simulink model "ALU_zipVer_Updated"  (R2023a)
settings: Solver=VariableStepAuto  StartTime=0.0  StopTime=10.0  RelTol=1e-3
settings Model: Creator=serge  LastModifiedBy=serge

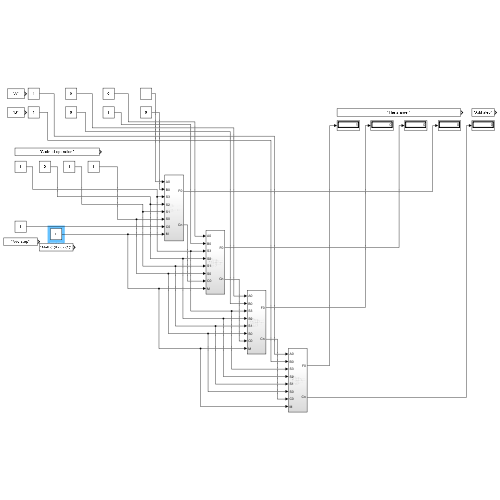
[thumbnail: Simulink's stored preview of the top-level diagram]
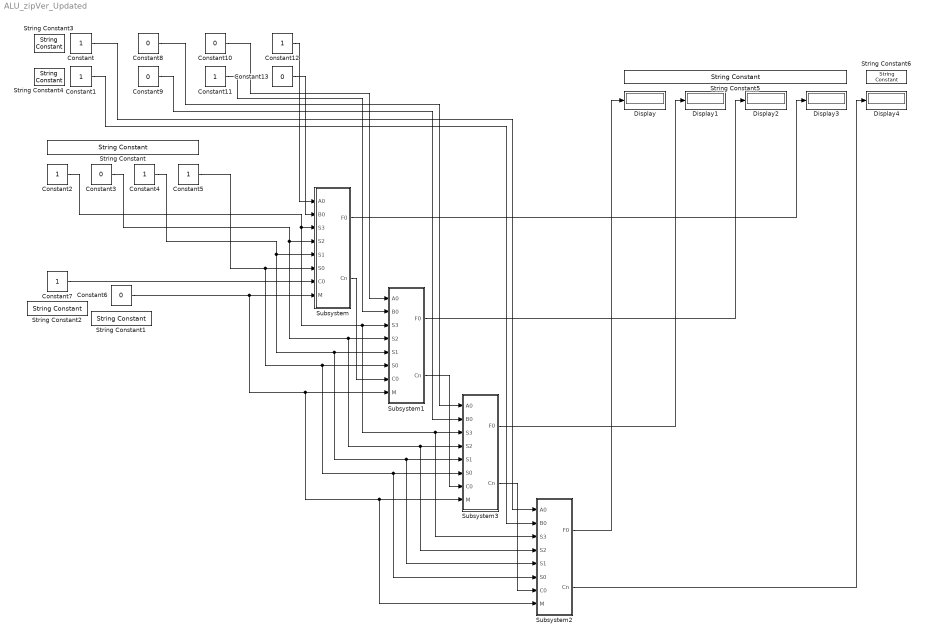
== system ALU_zipVer_Updated ==
  Constant{,1..2,4..5,7,11..12} (8 alike) : Constant
  Constant{3,6,8..10,13} (6 alike) : Constant  Value=0
  Display{,1..4} (5 alike) : Display
  String Constant : StringConstant  String="\"Code of operation\""
  String Constant1 : StringConstant  String="\"Math(0)/Logic(1)\""
  String Constant2 : StringConstant  String="\"Add step\""
  String Constant3 : StringConstant  String="\"A\""
  String Constant4 : StringConstant  String="\"B\""
  String Constant5 : StringConstant  String="\"The answer\""
  String Constant6 : StringConstant  String="\"Add step\""
  Subsystem : Subsystem
  Subsystem1 : Subsystem
  Subsystem2 : Subsystem
  Subsystem3 : Subsystem
  wires:
  Constant/1 -> Subsystem2/1(A0)
  Constant1/1 -> Subsystem2/2(B0)
  Constant3/1 -> Subsystem1/4(S2), Subsystem2/4(S2), Subsystem3/4(S2), Subsystem/4(S2)
  Constant4/1 -> Subsystem1/5(S1), Subsystem2/5(S1), Subsystem3/5(S1), Subsystem/5(S1)
  Constant5/1 -> Subsystem2/6(S0), Subsystem3/6(S0), Subsystem1/6(S0), Subsystem/6(S0)
  Constant6/1 -> Subsystem1/8(M), Subsystem2/8(M), Subsystem3/8(M), Subsystem/8(M)
  Constant7/1 -> Subsystem/7(C0)
  Subsystem/2(Cn) -> Subsystem1/7(C0)
  Subsystem1/2(Cn) -> Subsystem3/7(C0)
  Subsystem3/2(Cn) -> Subsystem2/7(C0)
  Constant2/1 -> Subsystem1/3(S3), Subsystem2/3(S3), Subsystem3/3(S3), Subsystem/3(S3)
  Constant8/1 -> Subsystem3/1(A0)
  Constant9/1 -> Subsystem3/2(B0)
  Constant10/1 -> Subsystem1/1(A0)
  Constant11/1 -> Subsystem1/2(B0)
  Constant13/1 -> Subsystem/2(B0)
  Constant12/1 -> Subsystem/1(A0)
  Subsystem2/2(Cn) -> Display4/1
  Subsystem2/1(F0) -> Display/1
  Subsystem3/1(F0) -> Display1/1
  Subsystem1/1(F0) -> Display2/1
  Subsystem/1(F0) -> Display3/1

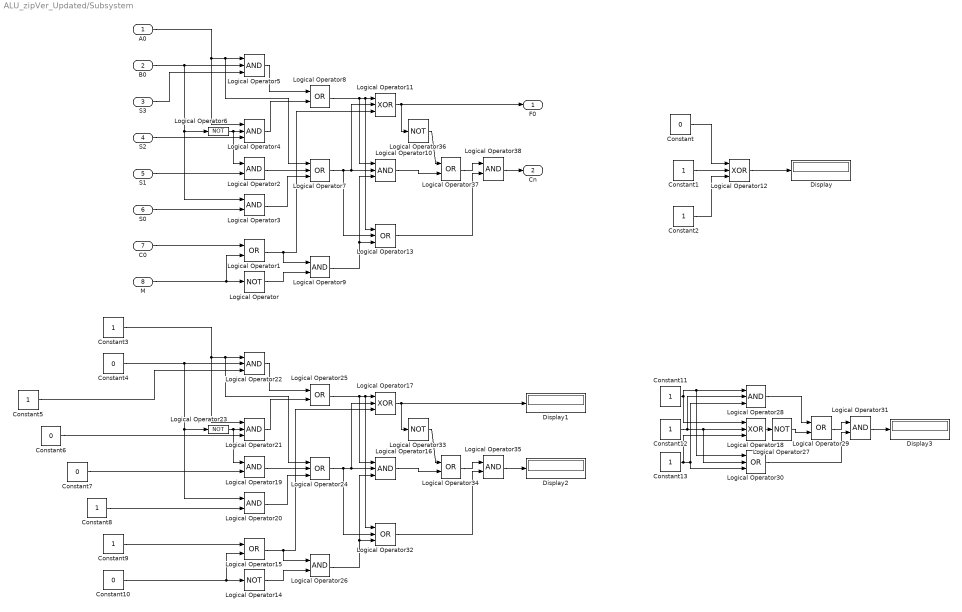
== system ALU_zipVer_Updated/Subsystem ==
  A0 : Inport
  B0 : Inport  Port=2
  S3 : Inport  Port=3
  S2 : Inport  Port=4
  S1 : Inport  Port=5
  S0 : Inport  Port=6
  C0 : Inport  Port=7
  M : Inport  Port=8
  Constant{,4,6..7,10} (5 alike) : Constant  Value=0
  Constant{1..3,5,8..9,11..13} (9 alike) : Constant
  Display{,1..3} (4 alike) : Display
  Logical Operator{,6,14,23} (4 alike) : Logic  Operator=NOT  AllPortsSameDT=off  OutDataTypeStr=boolean
  Logical Operator{1,8,15,25,29,34,37} (7 alike) : Logic  Operator=OR  AllPortsSameDT=off  OutDataTypeStr=boolean
  Logical Operator{4..5,10,16,21..22,28} (7 alike) : Logic  Inputs=3  AllPortsSameDT=off  OutDataTypeStr=boolean
  Logical Operator{11..12,17..18} (4 alike) : Logic  Operator=XOR  Inputs=3  AllPortsSameDT=off  OutDataTypeStr=boolean
  Logical Operator{7,13,24,30,32} (5 alike) : Logic  Operator=OR  Inputs=3  AllPortsSameDT=off  OutDataTypeStr=boolean
  Logical Operator{2..3,9,19..20,26,31,35,38} (9 alike) : Logic  AllPortsSameDT=off  OutDataTypeStr=boolean
  Logical Operator27 : Logic  Operator=NOT  Inputs=3  AllPortsSameDT=off  OutDataTypeStr=boolean
  Logical Operator33 : Logic  Operator=NOT  Inputs=3  AllPortsSameDT=off  OutDataTypeStr=boolean
  Logical Operator36 : Logic  Operator=NOT  Inputs=3  AllPortsSameDT=off  OutDataTypeStr=boolean
  F0 : Outport
  Cn : Outport  Port=2
  wires:
  S0/1 -> Logical Operator3/2
  Logical Operator6/1 -> Logical Operator2/1, Logical Operator4/2
  B0/1 -> Logical Operator5/2, Logical Operator6/1, Logical Operator3/1
  Logical Operator5/1 -> Logical Operator8/1
  Logical Operator/1 -> Logical Operator9/2
  M/1 -> Logical Operator/1, Logical Operator1/2
  A0/1 -> Logical Operator7/1, Logical Operator5/1, Logical Operator4/1
  S3/1 -> Logical Operator5/3
  C0/1 -> Logical Operator1/1
  Logical Operator4/1 -> Logical Operator8/2
  Logical Operator2/1 -> Logical Operator7/2
  Logical Operator3/1 -> Logical Operator7/3
  S1/1 -> Logical Operator2/2
  S2/1 -> Logical Operator4/3
  Constant/1 -> Logical Operator12/1
  Constant1/1 -> Logical Operator12/2
  Constant2/1 -> Logical Operator12/3
  Logical Operator12/1 -> Display/1
  Logical Operator25/1 -> Logical Operator16/1, Logical Operator32/1, Logical Operator17/1
  Logical Operator22/1 -> Logical Operator25/1
  Logical Operator21/1 -> Logical Operator25/2
  Constant6/1 -> Logical Operator21/3
  Constant9/1 -> Logical Operator15/1
  Logical Operator14/1 -> Logical Operator26/2
  Logical Operator26/1 -> Logical Operator32/3, Logical Operator16/3
  Constant3/1 -> Logical Operator24/1, Logical Operator22/1, Logical Operator21/1
  Constant4/1 -> Logical Operator22/2, Logical Operator23/1, Logical Operator20/1
  Logical Operator15/1 -> Logical Operator26/1, Logical Operator17/3
  Constant10/1 -> Logical Operator14/1, Logical Operator15/2
  Logical Operator24/1 -> Logical Operator32/2, Logical Operator17/2, Logical Operator16/2
  Logical Operator19/1 -> Logical Operator24/2
  Logical Operator16/1 -> Logical Operator34/2
  Constant8/1 -> Logical Operator20/2
  Logical Operator23/1 -> Logical Operator19/1, Logical Operator21/2
  Constant5/1 -> Logical Operator22/3
  Constant7/1 -> Logical Operator19/2
  Logical Operator20/1 -> Logical Operator24/3
  Logical Operator17/1 -> Logical Operator33/1, Display1/1
  Constant11/1 -> Logical Operator30/1, Logical Operator28/1, Logical Operator18/1
  Constant12/1 -> Logical Operator28/2, Logical Operator30/2, Logical Operator18/2
  Constant13/1 -> Logical Operator30/3, Logical Operator28/3, Logical Operator18/3
  Logical Operator18/1 -> Logical Operator27/1
  Logical Operator27/1 -> Logical Operator29/2
  Logical Operator28/1 -> Logical Operator29/1
  Logical Operator29/1 -> Logical Operator31/1
  Logical Operator30/1 -> Logical Operator31/2
  Logical Operator31/1 -> Display3/1
  Logical Operator33/1 -> Logical Operator34/1
  Logical Operator34/1 -> Logical Operator35/1
  Logical Operator32/1 -> Logical Operator35/2
  Logical Operator35/1 -> Display2/1
  Logical Operator8/1 -> Logical Operator10/1, Logical Operator13/1, Logical Operator11/1
  Logical Operator38/1 -> Cn/1
  Logical Operator10/1 -> Logical Operator37/2
  Logical Operator36/1 -> Logical Operator37/1
  Logical Operator37/1 -> Logical Operator38/1
  Logical Operator13/1 -> Logical Operator38/2
  Logical Operator11/1 -> F0/1, Logical Operator36/1
  Logical Operator1/1 -> Logical Operator11/3, Logical Operator9/1
  Logical Operator7/1 -> Logical Operator13/2, Logical Operator11/2, Logical Operator10/2
  Logical Operator9/1 -> Logical Operator13/3, Logical Operator10/3

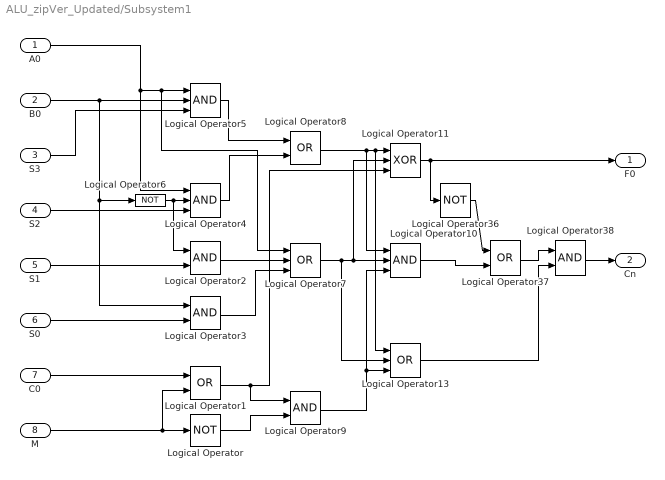
== system ALU_zipVer_Updated/Subsystem1 ==
  A0 : Inport
  B0 : Inport  Port=2
  S3 : Inport  Port=3
  S2 : Inport  Port=4
  S1 : Inport  Port=5
  S0 : Inport  Port=6
  C0 : Inport  Port=7
  M : Inport  Port=8
  Logical Operator : Logic  Operator=NOT  AllPortsSameDT=off  OutDataTypeStr=boolean
  Logical Operator1 : Logic  Operator=OR  AllPortsSameDT=off  OutDataTypeStr=boolean
  Logical Operator10 : Logic  Inputs=3  AllPortsSameDT=off  OutDataTypeStr=boolean
  Logical Operator11 : Logic  Operator=XOR  Inputs=3  AllPortsSameDT=off  OutDataTypeStr=boolean
  Logical Operator13 : Logic  Operator=OR  Inputs=3  AllPortsSameDT=off  OutDataTypeStr=boolean
  Logical Operator{2..3,9,38} (4 alike) : Logic  AllPortsSameDT=off  OutDataTypeStr=boolean
  Logical Operator36 : Logic  Operator=NOT  Inputs=3  AllPortsSameDT=off  OutDataTypeStr=boolean
  Logical Operator37 : Logic  Operator=OR  AllPortsSameDT=off  OutDataTypeStr=boolean
  Logical Operator4 : Logic  Inputs=3  AllPortsSameDT=off  OutDataTypeStr=boolean
  Logical Operator5 : Logic  Inputs=3  AllPortsSameDT=off  OutDataTypeStr=boolean
  Logical Operator6 : Logic  Operator=NOT  AllPortsSameDT=off  OutDataTypeStr=boolean
  Logical Operator7 : Logic  Operator=OR  Inputs=3  AllPortsSameDT=off  OutDataTypeStr=boolean
  Logical Operator8 : Logic  Operator=OR  AllPortsSameDT=off  OutDataTypeStr=boolean
  F0 : Outport
  Cn : Outport  Port=2
  wires:
  Logical Operator2/1 -> Logical Operator7/2
  Logical Operator4/1 -> Logical Operator8/2
  S2/1 -> Logical Operator4/3
  Logical Operator5/1 -> Logical Operator8/1
  Logical Operator36/1 -> Logical Operator37/1
  Logical Operator13/1 -> Logical Operator38/2
  Logical Operator37/1 -> Logical Operator38/1
  C0/1 -> Logical Operator1/1
  Logical Operator/1 -> Logical Operator9/2
  Logical Operator8/1 -> Logical Operator10/1, Logical Operator13/1, Logical Operator11/1
  Logical Operator7/1 -> Logical Operator13/2, Logical Operator11/2, Logical Operator10/2
  Logical Operator11/1 -> F0/1, Logical Operator36/1
  Logical Operator9/1 -> Logical Operator13/3, Logical Operator10/3
  A0/1 -> Logical Operator7/1, Logical Operator5/1, Logical Operator4/1
  B0/1 -> Logical Operator5/2, Logical Operator6/1, Logical Operator3/1
  Logical Operator1/1 -> Logical Operator11/3, Logical Operator9/1
  M/1 -> Logical Operator/1, Logical Operator1/2
  S0/1 -> Logical Operator3/2
  Logical Operator10/1 -> Logical Operator37/2
  Logical Operator6/1 -> Logical Operator2/1, Logical Operator4/2
  S3/1 -> Logical Operator5/3
  S1/1 -> Logical Operator2/2
  Logical Operator3/1 -> Logical Operator7/3
  Logical Operator38/1 -> Cn/1

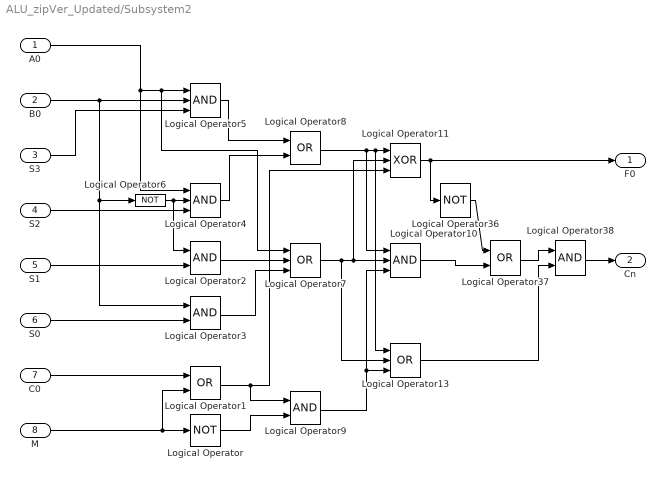
== system ALU_zipVer_Updated/Subsystem2 ==
  A0 : Inport
  B0 : Inport  Port=2
  S3 : Inport  Port=3
  S2 : Inport  Port=4
  S1 : Inport  Port=5
  S0 : Inport  Port=6
  C0 : Inport  Port=7
  M : Inport  Port=8
  Logical Operator : Logic  Operator=NOT  AllPortsSameDT=off  OutDataTypeStr=boolean
  Logical Operator1 : Logic  Operator=OR  AllPortsSameDT=off  OutDataTypeStr=boolean
  Logical Operator10 : Logic  Inputs=3  AllPortsSameDT=off  OutDataTypeStr=boolean
  Logical Operator11 : Logic  Operator=XOR  Inputs=3  AllPortsSameDT=off  OutDataTypeStr=boolean
  Logical Operator13 : Logic  Operator=OR  Inputs=3  AllPortsSameDT=off  OutDataTypeStr=boolean
  Logical Operator{2..3,9,38} (4 alike) : Logic  AllPortsSameDT=off  OutDataTypeStr=boolean
  Logical Operator36 : Logic  Operator=NOT  Inputs=3  AllPortsSameDT=off  OutDataTypeStr=boolean
  Logical Operator37 : Logic  Operator=OR  AllPortsSameDT=off  OutDataTypeStr=boolean
  Logical Operator4 : Logic  Inputs=3  AllPortsSameDT=off  OutDataTypeStr=boolean
  Logical Operator5 : Logic  Inputs=3  AllPortsSameDT=off  OutDataTypeStr=boolean
  Logical Operator6 : Logic  Operator=NOT  AllPortsSameDT=off  OutDataTypeStr=boolean
  Logical Operator7 : Logic  Operator=OR  Inputs=3  AllPortsSameDT=off  OutDataTypeStr=boolean
  Logical Operator8 : Logic  Operator=OR  AllPortsSameDT=off  OutDataTypeStr=boolean
  F0 : Outport
  Cn : Outport  Port=2
  wires:
  Logical Operator2/1 -> Logical Operator7/2
  Logical Operator4/1 -> Logical Operator8/2
  S2/1 -> Logical Operator4/3
  Logical Operator5/1 -> Logical Operator8/1
  Logical Operator36/1 -> Logical Operator37/1
  Logical Operator13/1 -> Logical Operator38/2
  Logical Operator37/1 -> Logical Operator38/1
  C0/1 -> Logical Operator1/1
  Logical Operator/1 -> Logical Operator9/2
  Logical Operator8/1 -> Logical Operator10/1, Logical Operator13/1, Logical Operator11/1
  Logical Operator7/1 -> Logical Operator13/2, Logical Operator11/2, Logical Operator10/2
  Logical Operator11/1 -> F0/1, Logical Operator36/1
  Logical Operator9/1 -> Logical Operator13/3, Logical Operator10/3
  A0/1 -> Logical Operator7/1, Logical Operator5/1, Logical Operator4/1
  B0/1 -> Logical Operator5/2, Logical Operator6/1, Logical Operator3/1
  Logical Operator1/1 -> Logical Operator11/3, Logical Operator9/1
  M/1 -> Logical Operator/1, Logical Operator1/2
  S0/1 -> Logical Operator3/2
  Logical Operator10/1 -> Logical Operator37/2
  Logical Operator6/1 -> Logical Operator2/1, Logical Operator4/2
  S3/1 -> Logical Operator5/3
  S1/1 -> Logical Operator2/2
  Logical Operator3/1 -> Logical Operator7/3
  Logical Operator38/1 -> Cn/1

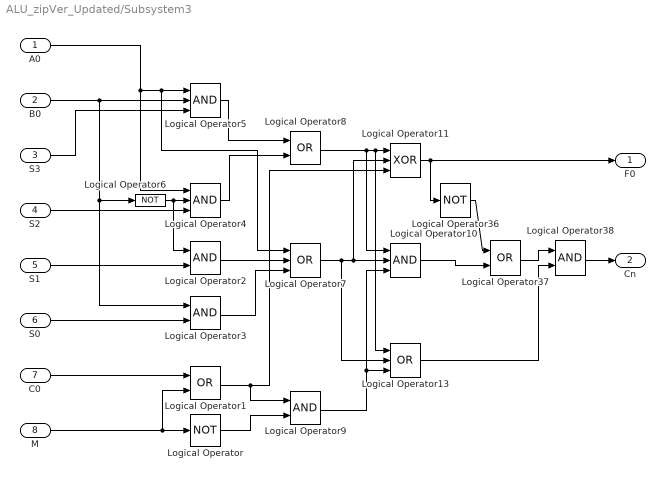
== system ALU_zipVer_Updated/Subsystem3 ==
  A0 : Inport
  B0 : Inport  Port=2
  S3 : Inport  Port=3
  S2 : Inport  Port=4
  S1 : Inport  Port=5
  S0 : Inport  Port=6
  C0 : Inport  Port=7
  M : Inport  Port=8
  Logical Operator : Logic  Operator=NOT  AllPortsSameDT=off  OutDataTypeStr=boolean
  Logical Operator1 : Logic  Operator=OR  AllPortsSameDT=off  OutDataTypeStr=boolean
  Logical Operator10 : Logic  Inputs=3  AllPortsSameDT=off  OutDataTypeStr=boolean
  Logical Operator11 : Logic  Operator=XOR  Inputs=3  AllPortsSameDT=off  OutDataTypeStr=boolean
  Logical Operator13 : Logic  Operator=OR  Inputs=3  AllPortsSameDT=off  OutDataTypeStr=boolean
  Logical Operator{2..3,9,38} (4 alike) : Logic  AllPortsSameDT=off  OutDataTypeStr=boolean
  Logical Operator36 : Logic  Operator=NOT  Inputs=3  AllPortsSameDT=off  OutDataTypeStr=boolean
  Logical Operator37 : Logic  Operator=OR  AllPortsSameDT=off  OutDataTypeStr=boolean
  Logical Operator4 : Logic  Inputs=3  AllPortsSameDT=off  OutDataTypeStr=boolean
  Logical Operator5 : Logic  Inputs=3  AllPortsSameDT=off  OutDataTypeStr=boolean
  Logical Operator6 : Logic  Operator=NOT  AllPortsSameDT=off  OutDataTypeStr=boolean
  Logical Operator7 : Logic  Operator=OR  Inputs=3  AllPortsSameDT=off  OutDataTypeStr=boolean
  Logical Operator8 : Logic  Operator=OR  AllPortsSameDT=off  OutDataTypeStr=boolean
  F0 : Outport
  Cn : Outport  Port=2
  wires:
  Logical Operator2/1 -> Logical Operator7/2
  Logical Operator4/1 -> Logical Operator8/2
  S2/1 -> Logical Operator4/3
  Logical Operator5/1 -> Logical Operator8/1
  Logical Operator36/1 -> Logical Operator37/1
  Logical Operator13/1 -> Logical Operator38/2
  Logical Operator37/1 -> Logical Operator38/1
  C0/1 -> Logical Operator1/1
  Logical Operator/1 -> Logical Operator9/2
  Logical Operator8/1 -> Logical Operator10/1, Logical Operator13/1, Logical Operator11/1
  Logical Operator7/1 -> Logical Operator13/2, Logical Operator11/2, Logical Operator10/2
  Logical Operator11/1 -> F0/1, Logical Operator36/1
  Logical Operator9/1 -> Logical Operator13/3, Logical Operator10/3
  A0/1 -> Logical Operator7/1, Logical Operator5/1, Logical Operator4/1
  B0/1 -> Logical Operator5/2, Logical Operator6/1, Logical Operator3/1
  Logical Operator1/1 -> Logical Operator11/3, Logical Operator9/1
  M/1 -> Logical Operator/1, Logical Operator1/2
  S0/1 -> Logical Operator3/2
  Logical Operator10/1 -> Logical Operator37/2
  Logical Operator6/1 -> Logical Operator2/1, Logical Operator4/2
  S3/1 -> Logical Operator5/3
  S1/1 -> Logical Operator2/2
  Logical Operator3/1 -> Logical Operator7/3
  Logical Operator38/1 -> Cn/1
